simulink model "HumidifierController_Start"  (R2025b)
settings: Solver=VariableStepAuto  StartTime=0.0  StopTime=inf  FixedStep=0.05  RelTol=1e-3
PreLoadFcn:
  | load rel_humidity.mat;
  | load rel_humidity_heatedwire.mat;
  | load rel_humidityInput.mat;
settings Model: DataDictionary=Humidifier_Logical_Start.sldd  Creator=ppatel  LastModifiedBy=ppatel

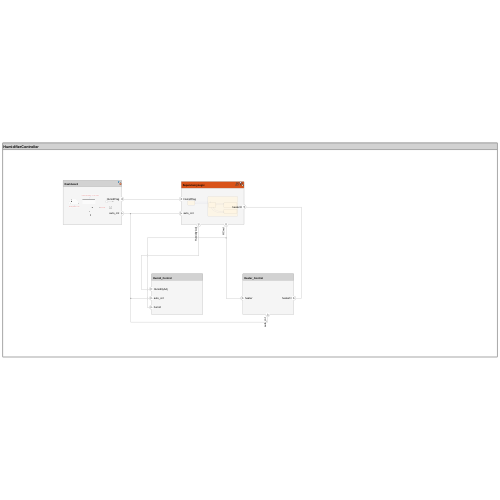
[thumbnail: Simulink's stored preview of the top-level diagram]
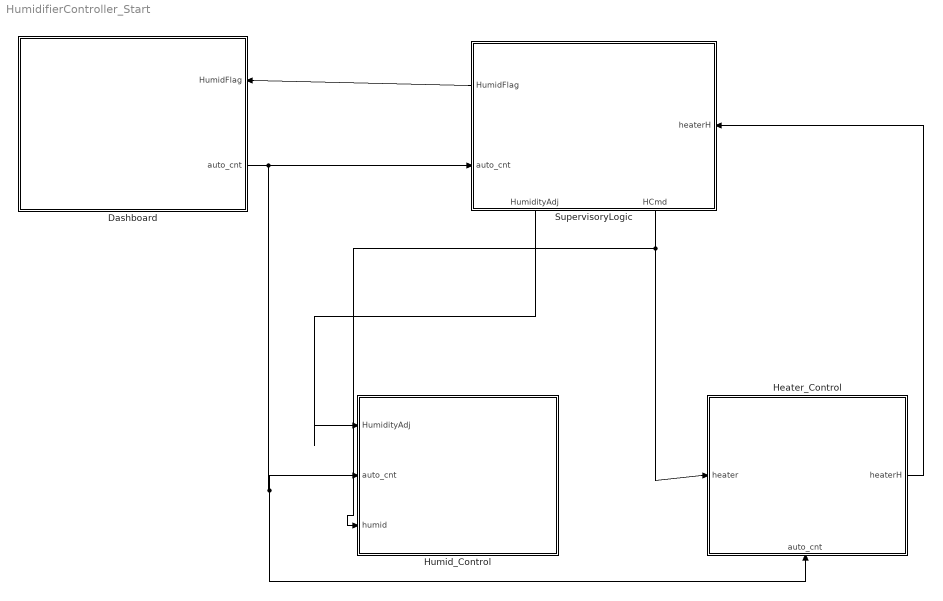
== system HumidifierController_Start ==
  Dashboard : Subsystem
      settings: PortSchema="{\"entries\":[{\"content\":{\"headerSize\":26,\"margin\":15,\"minimumSpacing\":25,\"sides\":[{\"content\":{},\"type\":\"ConnectorPlacement.EquallySpacedRectSide\",\"uuid\":\"18e365e9-4ccc-4943-ae85-7abdeaed82a1\"},{\"content\":{\"connectorIds\":[\"In1\",\"Out1\"],\"side\":\"RIGHT\"},\"type\":\"ConnectorPlacement.EquallySpacedRectSide\",\"uuid\":\"aafe069d-304d-4de7-a3f2-52986cc58723\"},{\"content\":{\"side\":\"TOP\"},\"type\":\"ConnectorPlacement.EquallySpacedRectSide\",\"uuid\":\"efebfcde-c43f-4485-9584-5cc34f249b53\"}]},\"type\":\"ConnectorPlacement.EquallySpacedConnector\",\"uuid\":\"82b97aa5-a7bf-41ea-90eb-26c45b3d9e14\"}],\"packageUris\":[\"http://schema.mathworks.com/mf0/Connector/R2020b\"],\"version\":\"1.0\"}"
  Heater_Control : Subsystem
      settings: PortSchema="{\"entries\":[{\"content\":{\"headerSize\":26,\"margin\":15,\"minimumSpacing\":25,\"sides\":[{\"content\":{\"connectorIds\":[\"In2\"]},\"type\":\"ConnectorPlacement.EquallySpacedRectSide\",\"uuid\":\"99e36875-734e-4284-a16d-0dd8329bb214\"},{\"content\":{\"connectorIds\":[\"Out1\"],\"side\":\"RIGHT\"},\"type\":\"ConnectorPlacement.EquallySpacedRectSide\",\"uuid\":\"0324b7e5-1355-4e51-a01a-8e9c05dd1998\"},{\"content\":{\"side\":\"TOP\"},\"type\":\"ConnectorPlacement.EquallySpacedRectSide\",\"uuid\":\"4a4ee909-e0de-438a-a471-b08fa4bad9c1\"},{\"content\":{\"connectorIds\":[\"In1\"],\"side\":\"BOTTOM\"},\"type\":\"ConnectorPlacement.EquallySpacedRectSide\",\"uuid\":\"24dcbc3f-ea65-4cef-9c7f-3514e7bc5c11\"}]},\"type\":\"ConnectorPlacement.EquallySpacedConnector\",\"uuid\":\"54df2e5e-59bf-4d38-9901-d21c896100d7\"}],\"packageUris\":[\"http://schema.mathworks.com/mf0/Connector/R2020b\"],\"version\":\"1.0\"}"
  Humid_Control : Subsystem
      settings: PortSchema="{\"entries\":[{\"content\":{\"headerSize\":26,\"margin\":15,\"minimumSpacing\":25,\"sides\":[{\"content\":{\"connectorIds\":[\"In1\",\"In2\",\"In3\"]},\"type\":\"ConnectorPlacement.EquallySpacedRectSide\",\"uuid\":\"99e36875-734e-4284-a16d-0dd8329bb214\"},{\"content\":{\"side\":\"RIGHT\"},\"type\":\"ConnectorPlacement.EquallySpacedRectSide\",\"uuid\":\"0324b7e5-1355-4e51-a01a-8e9c05dd1998\"},{\"content\":{\"side\":\"TOP\"},\"type\":\"ConnectorPlacement.EquallySpacedRectSide\",\"uuid\":\"4a4ee909-e0de-438a-a471-b08fa4bad9c1\"}]},\"type\":\"ConnectorPlacement.EquallySpacedConnector\",\"uuid\":\"54df2e5e-59bf-4d38-9901-d21c896100d7\"}],\"packageUris\":[\"http://schema.mathworks.com/mf0/Connector/R2020b\"],\"version\":\"1.0\"}"
  SupervisoryLogic : Stateflow chart  TreatAsAtomicUnit=on
      settings: PortSchema="{\"entries\":[{\"content\":{\"headerSize\":26,\"margin\":15,\"minimumSpacing\":25,\"sides\":[{\"content\":{\"connectorIds\":[\"Out2\",\"In1\"]},\"type\":\"ConnectorPlacement.EquallySpacedRectSide\",\"uuid\":\"18e365e9-4ccc-4943-ae85-7abdeaed82a1\"},{\"content\":{\"connectorIds\":[\"In2\"],\"side\":\"RIGHT\"},\"type\":\"ConnectorPlacement.EquallySpacedRectSide\",\"uuid\":\"aafe069d-304d-4de7-a3f2-52986cc58723\"},{\"content\":{\"side\":\"TOP\"},\"type\":\"ConnectorPlacement.EquallySpacedRectSide\",\"uuid\":\"efebfcde-c43f-4485-9584-5cc34f249b53\"},{\"content\":{\"connectorIds\":[\"Out3\",\"Out1\"],\"side\":\"BOTTOM\"},\"type\":\"ConnectorPlacement.EquallySpacedRectSide\",\"uuid\":\"e6545cc7-72fb-4675-8982-3f6edbb72f82\"}]},\"type\":\"ConnectorPlacement.EquallySpacedConnector\",\"uuid\":\"82b97aa5-a7bf-41ea-90eb-26c45b3d9e14\"}],\"packageUris\":[\"http://schema.mathworks.com/mf0/Connector/R2020b\"],\"version\":\"1.0\"}"
  wires:
  Dashboard/1(auto_cnt) -> Heater_Control/1(auto_cnt), Humid_Control/2(auto_cnt), SupervisoryLogic/1(auto_cnt)
  SupervisoryLogic/1(HCmd) -> Heater_Control/2(heater), Humid_Control/3(humid)
  SupervisoryLogic/2(HumidFlag) -> Dashboard/1(HumidFlag)
  SupervisoryLogic/3(HumidityAdj) -> Humid_Control/1(HumidityAdj)
  Heater_Control/1(heaterH) -> SupervisoryLogic/2(heaterH)

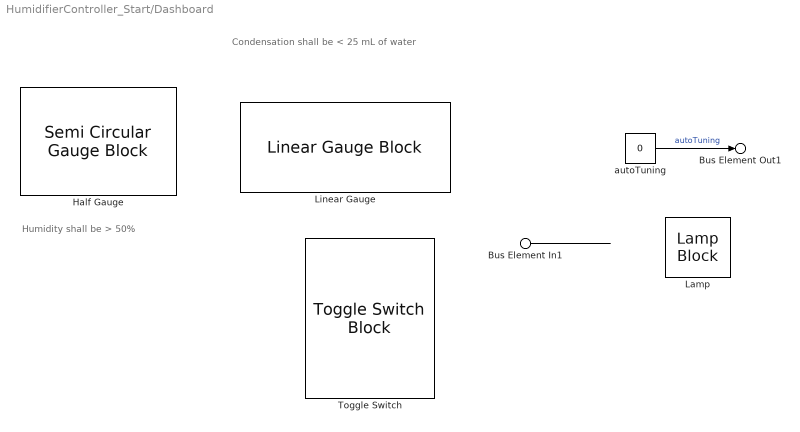
== system HumidifierController_Start/Dashboard ==
  note: Condensation shall be < 25 mL of water
  note: Humidity shall be > 50%
  Bus Element In1 : Inport  PortName=HumidFlag
  Half Gauge : SemiCircularGaugeBlock  TickInterval=25  FontColor=[0.0, 0.0, 0.0]
  Lamp : LampBlock  LabelPosition=Hide  DefaultColor=[192.0, 192.0, 192.0]
  Linear Gauge : LinearGaugeBlock  ScaleMax=50  FontColor=[0.0, 0.0, 0.0]
  Toggle Switch : ToggleSwitchBlock
  autoTuning : Constant  Value=0
  Bus Element Out1 : Outport  PortName=auto_cnt
  wires:
  autoTuning/1 -> Bus Element Out1/1  "autoTuning"
  Bus Element In1/1 -> ?

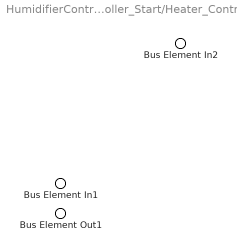
== system HumidifierController_Start/Heater_Control ==
  Bus Element In2 : Inport  PortName=auto_cnt
  Bus Element In1 : Inport  Port=2  PortName=heater
  Bus Element Out1 : Outport  PortName=heaterH

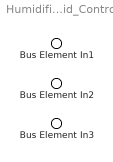
== system HumidifierController_Start/Humid_Control ==
  Bus Element In1 : Inport  PortName=HumidityAdj
  Bus Element In2 : Inport  Port=2  PortName=auto_cnt
  Bus Element In3 : Inport  Port=3  PortName=humid

== stateflow chart HumidifierController_Start/SupervisoryLogic ==
  state Auto_Control
    en:
    HCmd.Humidity = 20;
    HCmd.Heater = 0;
    HumidFlag = true;
    state no_change
      en:
      HumidityAdj.data = false;
      send(HumidityAdj);
    state HumidControl
      en:
      HCmd.Humidity = HCmd.Humidity + 5;
      HumidityAdj.data = true;
      send(HumidityAdj);
    state HeaterControl
      en:
      HCmd.Heater = HCmd.Heater + 5;
    (default) -> no_change
    no_change -> HumidControl [order 1] : [heaterH.Insp_Humidity < 50]
    HumidControl -> no_change : after(3,sec)
    no_change -> HeaterControl [order 2] : [heaterH.CondLvl > 25]
    HeaterControl -> no_change : after(1,sec)
  state Manual_Control
    en:
    HCmd.Humidity = 0;
    HCmd.Heater = 0;
    HumidFlag = false;
  (default) -> Manual_Control
  Manual_Control -> Auto_Control : [auto_cnt ==1]
  Auto_Control -> Manual_Control : [auto_cnt ==0]
  data: auto_cnt input; heaterH input Bus: Humidity; HCmd output Bus: Command; HumidFlag output; HumidityAdj output
